simulink model "verify_EU_Tapping_mdl"  (R2016b)
settings: Solver=ode45  StartTime=0.0  StopTime=24*3600  MaxStep=10  RelTol=1e-3  EnableMultiTasking=on
libraries: carnot x6
settings Model: Creator=drhf  LastModifiedBy=drhf
settings DataIOCC: LimitDataPoints=on  MaxDataPoints=1  SaveFormat=Array  SignalLoggingSaveFormat=ModelDataLogs
settings OptimizationCC: ExpressionDepthLimit=2147483647  LifeSpan=inf
settings DebuggingCC: UnderspecifiedInitializationDetection=Classic  MergeDetectMultiDrivingBlocksExec=none  SolverPrmCheckMsg=warning  StateNameClashWarn=warning  SFUnexpectedBacktrackingDiag=warning  SFNoUnconditionalDefaultTransitionDiag=warning  SFExecutionAtInitializationDiag=none
settings HardwareCC: ProdBitPerPointer=32  ProdBitPerSizeT=32  ProdBitPerPtrDiffT=32  ProdLargestAtomicFloat=None  ProdIntDivRoundTo=Undefined  ProdEndianess=Unspecified  ProdWordSize=32  ProdHWDeviceType=32-bit Generic
settings ModelReferenceCC: PropagateSignalLabelsOutOfModel=off
settings GRTTargetCC: TargetLangStandard=C89/C90 (ANSI)  GeneratePreprocessorConditionals=Disable all  CombineOutputUpdateFcns=off  GRTInterface=on
settings ConfigComp: CovMetricSettings=dw  CovHtmlReporting=on  CovSaveCumulativeToWorkspaceVar=on  CovSaveSingleToWorkspaceVar=on  CovExternalEMLEnable=off

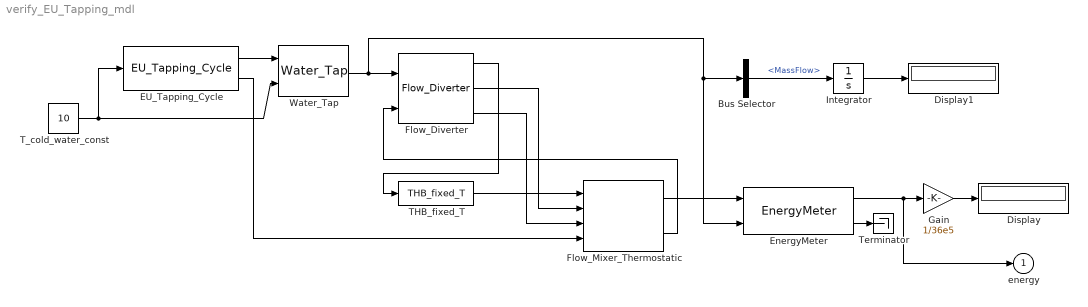
== system verify_EU_Tapping_mdl ==
  Bus Selector : BusSelector  OutputSignals=MassFlow
  Display : Display
  Display1 : Display
  EU_Tapping_Cycle : carnot/Load/Hot_Water_Tapping/EU_Tapping_Cycle  eu_tap=3XS
  EnergyMeter : carnot/Control/EnergyMeter
  Flow_Diverter : carnot/Hydraulics/Flow_Diverter
  Flow_Mixer_Thermostatic : carnot/Hydraulics/Flow_Mixer_Thermostatic  t=10
  Gain : Gain  Gain=1/36e5
  Integrator : Integrator
  THB_fixed_T : carnot/Source/Simple/THB_fixed_T  t=60
  T_cold_water_const : Constant  Value=10
  Terminator : Terminator
  Water_Tap : carnot/Load/Hot_Water_Tapping/Water_Tap  dia=0.02  p=2e5
  energy : Outport  InitialOutput=0
  wires:
  EnergyMeter/1 -> Gain/1, energy/1
  Gain/1 -> Display/1
  Water_Tap/1 -> Bus Selector/1, EnergyMeter/2, Flow_Diverter/1
  T_cold_water_const/1 -> EU_Tapping_Cycle/1, Water_Tap/2
  EU_Tapping_Cycle/1 -> Water_Tap/1
  EU_Tapping_Cycle/2 -> Flow_Mixer_Thermostatic/4
  Flow_Diverter/3 -> Flow_Mixer_Thermostatic/3
  Flow_Diverter/2 -> Flow_Mixer_Thermostatic/2
  THB_fixed_T/1 -> Flow_Mixer_Thermostatic/1
  Flow_Mixer_Thermostatic/1 -> EnergyMeter/1
  Flow_Mixer_Thermostatic/2 -> Flow_Diverter/2
  Flow_Diverter/1 -> THB_fixed_T/1
  Bus Selector/1 -> Integrator/1  "<MassFlow>"
  Integrator/1 -> Display1/1
  EnergyMeter/2 -> Terminator/1
